simulink model "simulate_battery_w_cap"  (R2021a)
settings: Solver=VariableStepAuto  StartTime=0.0  StopTime=time_val  RelTol=1e-3
settings Model: Creator=saleh  LastModifiedBy=saleh

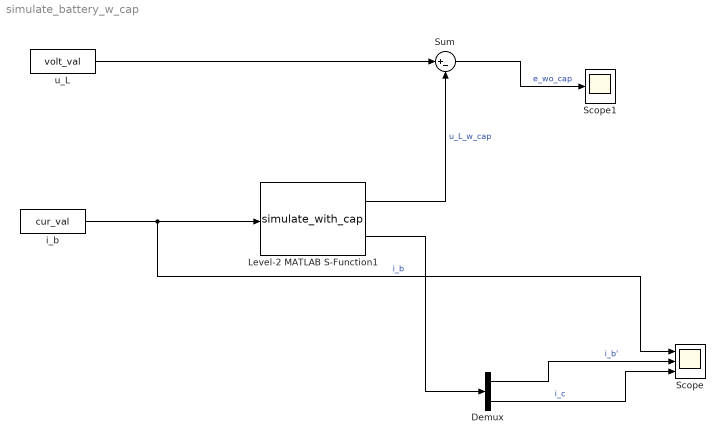
== system simulate_battery_w_cap ==
  Demux : Demux  Outputs=2
  Level-2 MATLAB S-Function1 : M-S-Function  FunctionName=simulate_with_cap  Parameters=x_conv, a, Qe, Cg
  Scope : Scope  NumInputPorts=3
  Scope1 : Scope
  Sum : Sum  Inputs=|+-
  i_b : FromWorkspace  VariableName=cur_val
  u_L : FromWorkspace  VariableName=volt_val
  wires:
  i_b/1 -> Scope/1, Level-2 MATLAB S-Function1/1  "i_b"
  Level-2 MATLAB S-Function1/2 -> Demux/1
  Demux/2 -> Scope/3  "i_c"
  Demux/1 -> Scope/2  "i_b'"
  u_L/1 -> Sum/1
  Level-2 MATLAB S-Function1/1 -> Sum/2  "u_L_w_cap"
  Sum/1 -> Scope1/1  "e_wo_cap"
